simulink model "MatlabFunctionBlock"  (R2022b)
settings: Solver=VariableStepAuto  StartTime=0.0  StopTime=10.0  RelTol=1e-3
settings Model: Creator=uditpant  LastModifiedBy=uditpant

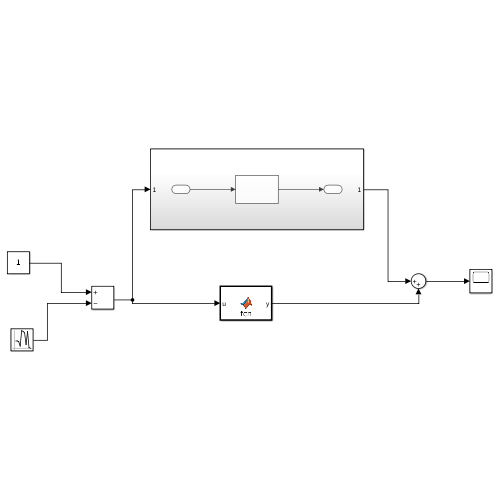
[thumbnail: Simulink's stored preview of the top-level diagram]
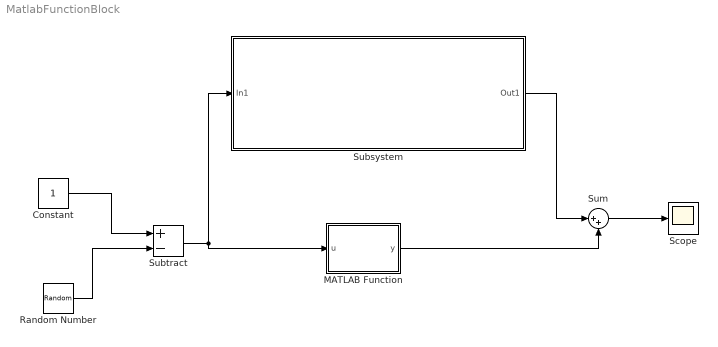
== system MatlabFunctionBlock ==
  Constant : Constant
  MATLAB Function : MATLAB Function  TreatAsAtomicUnit=on
  Random Number : RandomNumber  SampleTime=0.1
  Scope : Scope
  Subsystem : Subsystem
  Subtract : Sum  Inputs=+-
  Sum : Sum  Inputs=|++
  wires:
  Constant/1 -> Subtract/1
  Random Number/1 -> Subtract/2
  Subtract/1 -> MATLAB Function/1(u), Subsystem/1(In1)
  Subsystem/1(Out1) -> Sum/1
  MATLAB Function/1(y) -> Sum/2
  Sum/1 -> Scope/1

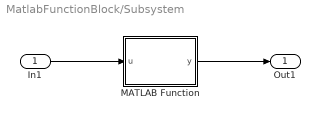
== system MatlabFunctionBlock/Subsystem ==
  In1 : Inport
  MATLAB Function : MATLAB Function  TreatAsAtomicUnit=on
  Out1 : Outport
  wires:
  In1/1 -> MATLAB Function/1(u)
  MATLAB Function/1(y) -> Out1/1

== matlab function MatlabFunctionBlock/MATLAB Function ==
  data: u input; y output
function y = fcn(u)
u = abs(u);
y = nthroot(u*u + 2*u, u*u);

== matlab function MatlabFunctionBlock/Subsystem/MATLAB Function ==
  data: u input; y output
function y = fcn(u)

y = sqrt(u*u + 2*u + 6);
